simulink model "DFADAS2_SenFus_v1_201204RC_training_210115"  (R2018b)
settings: Solver=FixedStepDiscrete  StartTime=0.0  StopTime=inf  FixedStep=0.002  RelTol=1e-3  EnableMultiTasking=on
PreLoadFcn:
  | RTWConfigurationCB('preloadfcn', bdroot);
libraries: canmsglib x108, simulink x48, canfdmsglib x12
(part 27 of 28)

== system DFADAS2_SenFus_v1_201204RC_training_210115/Signal Input (Input)/Signal Input (10ms) (Input10)/VehInfo/Body Electric System State Receive and Processing (BESRx)/Steering Lamp CAN Frame PreProcess (StLampCANFrmPPrcs)/CAN Diagnosis (CANDia)/CheckSum Diagnosis (ChkSumDia)/Bit Check(BChk)/Bit Operating (BOp) ==
  note: CheckSum Error Flag Discription:
      | 1 : Fault
      | 0 : Normal
  note: Checksum Preprocess -- ChksumPre
  BOp_bByte0 : Inport
  BOp_bByte1 : Inport  Port=2
  BOp_bByte2 : Inport  Port=3
  BOp_bByte3 : Inport  Port=4
  BOp_bByte4 : Inport  Port=5
  BOp_bByte5 : Inport  Port=6
  BOp_bByte6 : Inport  Port=7
  BOp_bByte7 : Inport  Port=8
  Add : Sum  Inputs=+++++++
  Add1 : Sum  Inputs=+-
  Add2 : Sum  Inputs=+-
  ChksumPre1 : Subsystem
  ChksumPre2 : Subsystem
  ChksumPre3 : Subsystem
  ChksumPre4 : Subsystem
  ChksumPre5 : Subsystem
  ChksumPre6 : Subsystem
  ChksumPre7 : Subsystem
  Constant : Constant  Value=256  OutDataTypeStr=uint16  SampleTime=-1
  Constant1 : Constant  Value=255  OutDataTypeStr=uint8  SampleTime=-1
  Constant2 : Constant  OutDataTypeStr=uint8  SampleTime=-1
  Constant3 : Constant  Value=0  OutDataTypeStr=uint8  SampleTime=-1
  Data Type Conversion6 : DataTypeConversion  OutDataTypeStr=uint8
  Math Function : Math  Operator=mod  OutputSignalType=real  SaturateOnIntegerOverflow=on
  Switch : Switch  Criteria=u2 ~= 0
  BOp_efChkSumErrFlg : Outport
  wires:
  Switch/1 -> BOp_efChkSumErrFlg/1
  Constant3/1 -> Switch/3
  Constant2/1 -> Switch/1
  BOp_bByte7/1 -> ChksumPre7/1(In1)
  ChksumPre7/1(Out1) -> Add/7
  ChksumPre6/1(Out1) -> Add/6
  BOp_bByte6/1 -> ChksumPre6/2(In2)
  BOp_bByte5/1 -> ChksumPre6/1(In1)
  ChksumPre5/1(Out1) -> Add/5
  BOp_bByte4/1 -> ChksumPre5/2(In2)
  BOp_bByte3/1 -> ChksumPre5/1(In1)
  ChksumPre4/1(Out1) -> Add/4
  BOp_bByte2/1 -> ChksumPre4/1(In1), ChksumPre3/1(In1), ChksumPre2/1(In1)
  ChksumPre1/1(Out1) -> Add/1
  BOp_bByte1/1 -> ChksumPre1/1(In1)
  Constant1/1 -> Add1/1
  Math Function/1 -> Data Type Conversion6/1
  Constant/1 -> Math Function/2
  Add/1 -> Math Function/1
  Data Type Conversion6/1 -> Add1/2
  ChksumPre2/1(Out1) -> Add/2
  ChksumPre3/1(Out1) -> Add/3
  BOp_bByte0/1 -> Add2/1
  Add1/1 -> Add2/2
  Add2/1 -> Switch/2

== system DFADAS2_SenFus_v1_201204RC_training_210115/Signal Input (Input)/Signal Input (10ms) (Input10)/VehInfo/Function Keys State Receive and Processing (FKeyStRx)/Key Enable CAN Frame PreProcess (KeyEnaCANFrmPPrcs)/CAN Diagnosis (CANDia)/CheckSum Diagnosis (ChkSumDia)/Bit Check(BChk)/Bit Operating (BOp) ==
  note: Checksum Preprocess -- ChksumPre
  note: CheckSum Error Flag Discription:
      | 1 : Fault
      | 0 : Normal
  BOp_bByte0 : Inport
  BOp_bByte1 : Inport  Port=2
  BOp_bByte2 : Inport  Port=3
  BOp_bByte3 : Inport  Port=4
  BOp_bByte4 : Inport  Port=5
  BOp_bByte5 : Inport  Port=6
  BOp_bByte6 : Inport  Port=7
  BOp_bByte7 : Inport  Port=8
  Add : Sum  Inputs=+++++++
  Add1 : Sum  Inputs=+-
  Add2 : Sum  Inputs=+-
  ChksumPre1 : Subsystem
  ChksumPre2 : Subsystem
  ChksumPre3 : Subsystem
  ChksumPre4 : Subsystem
  ChksumPre5 : Subsystem
  ChksumPre6 : Subsystem
  ChksumPre7 : Subsystem
  Constant : Constant  Value=256  OutDataTypeStr=uint16  SampleTime=-1
  Constant1 : Constant  Value=255  OutDataTypeStr=uint8  SampleTime=-1
  Constant2 : Constant  OutDataTypeStr=uint8  SampleTime=-1
  Constant3 : Constant  Value=0  OutDataTypeStr=uint8  SampleTime=-1
  Data Type Conversion6 : DataTypeConversion  OutDataTypeStr=uint8
  Math Function : Math  Operator=mod  OutputSignalType=real  SaturateOnIntegerOverflow=on
  Switch : Switch  Criteria=u2 ~= 0
  BOp_efChkSumErrFlg : Outport
  wires:
  Add2/1 -> Switch/2
  Add1/1 -> Add2/2
  BOp_bByte0/1 -> Add2/1
  ChksumPre3/1(Out1) -> Add/3
  ChksumPre2/1(Out1) -> Add/2
  Data Type Conversion6/1 -> Add1/2
  Add/1 -> Math Function/1
  Constant/1 -> Math Function/2
  Math Function/1 -> Data Type Conversion6/1
  Constant1/1 -> Add1/1
  BOp_bByte1/1 -> ChksumPre1/1(In1)
  ChksumPre1/1(Out1) -> Add/1
  BOp_bByte2/1 -> ChksumPre2/1(In1), ChksumPre3/1(In1), ChksumPre4/1(In1)
  ChksumPre4/1(Out1) -> Add/4
  BOp_bByte3/1 -> ChksumPre5/1(In1)
  BOp_bByte4/1 -> ChksumPre5/2(In2)
  ChksumPre5/1(Out1) -> Add/5
  BOp_bByte5/1 -> ChksumPre6/1(In1)
  BOp_bByte6/1 -> ChksumPre6/2(In2)
  ChksumPre6/1(Out1) -> Add/6
  ChksumPre7/1(Out1) -> Add/7
  BOp_bByte7/1 -> ChksumPre7/1(In1)
  Constant2/1 -> Switch/1
  Constant3/1 -> Switch/3
  Switch/1 -> BOp_efChkSumErrFlg/1

== system DFADAS2_SenFus_v1_201204RC_training_210115/Signal Input (Input)/Signal Input (10ms) (Input10)/VehInfo/MP5 Signal Receive (MP5Rx)1/CAN Diagnosis (CANDia)/CheckSum Diagnosis (ChkSumDia)/Bit Check(BChk)/Bit Operating (BOp)/ChksumPre1 ==
  In1 : Inport
  Data Type Conversion7 : DataTypeConversion  OutDataTypeStr=uint16
  Out1 : Outport
  wires:
  Data Type Conversion7/1 -> Out1/1
  In1/1 -> Data Type Conversion7/1

== system DFADAS2_SenFus_v1_201204RC_training_210115/Signal Input (Input)/Signal Input (10ms) (Input10)/VehInfo/MP5 Signal Receive (MP5Rx)1/CAN Diagnosis (CANDia)/CheckSum Diagnosis (ChkSumDia)/Bit Check(BChk)/Bit Operating (BOp)/ChksumPre2 ==
  In1 : Inport
  Data Type Conversion7 : DataTypeConversion  OutDataTypeStr=uint16
  Extract Bits : simulink/Logic and Bit Operations/Extract Bits  bitsToExtract=Range of bits  numBits=8  bitIdxRange=6  outScalingMode=Treat bit field as an integer
      settings: SourceProductName=Simulink
  Out1 : Outport
  wires:
  Extract Bits/1 -> Data Type Conversion7/1
  In1/1 -> Extract Bits/1
  Data Type Conversion7/1 -> Out1/1

== system DFADAS2_SenFus_v1_201204RC_training_210115/Signal Input (Input)/Signal Input (10ms) (Input10)/VehInfo/MP5 Signal Receive (MP5Rx)1/CAN Diagnosis (CANDia)/CheckSum Diagnosis (ChkSumDia)/Bit Check(BChk)/Bit Operating (BOp)/ChksumPre3 ==
  In1 : Inport
  Data Type Conversion8 : DataTypeConversion  OutDataTypeStr=uint16
  Extract Bits1 : simulink/Logic and Bit Operations/Extract Bits  bitsToExtract=Range of bits  numBits=8  bitIdxRange=5  outScalingMode=Treat bit field as an integer
      settings: SourceProductName=Simulink
  Out1 : Outport
  wires:
  Extract Bits1/1 -> Data Type Conversion8/1
  In1/1 -> Extract Bits1/1
  Data Type Conversion8/1 -> Out1/1

== system DFADAS2_SenFus_v1_201204RC_training_210115/Signal Input (Input)/Signal Input (10ms) (Input10)/VehInfo/MP5 Signal Receive (MP5Rx)1/CAN Diagnosis (CANDia)/CheckSum Diagnosis (ChkSumDia)/Bit Check(BChk)/Bit Operating (BOp)/ChksumPre4 ==
  In1 : Inport
  Data Type Conversion8 : DataTypeConversion  OutDataTypeStr=uint16
  Extract Bits1 : simulink/Logic and Bit Operations/Extract Bits  bitsToExtract=Range of bits  numBits=8  bitIdxRange=4  outScalingMode=Treat bit field as an integer
      settings: SourceProductName=Simulink
  Out1 : Outport
  wires:
  Data Type Conversion8/1 -> Out1/1
  In1/1 -> Extract Bits1/1
  Extract Bits1/1 -> Data Type Conversion8/1

== system DFADAS2_SenFus_v1_201204RC_training_210115/Signal Input (Input)/Signal Input (10ms) (Input10)/VehInfo/MP5 Signal Receive (MP5Rx)1/CAN Diagnosis (CANDia)/CheckSum Diagnosis (ChkSumDia)/Bit Check(BChk)/Bit Operating (BOp)/ChksumPre5 ==
  In1 : Inport
  In2 : Inport  Port=2
  Add : Sum
  Data Type Conversion1 : DataTypeConversion  OutDataTypeStr=uint16
  Data Type Conversion4 : DataTypeConversion  OutDataTypeStr=uint16
  Shift Arithmetic2 : ArithShift  BitShiftNumber=-8
  Out1 : Outport
  wires:
  Data Type Conversion1/1 -> Add/2
  Data Type Conversion4/1 -> Shift Arithmetic2/1
  Add/1 -> Out1/1
  Shift Arithmetic2/1 -> Add/1
  In2/1 -> Data Type Conversion1/1
  In1/1 -> Data Type Conversion4/1

== system DFADAS2_SenFus_v1_201204RC_training_210115/Signal Input (Input)/Signal Input (10ms) (Input10)/VehInfo/MP5 Signal Receive (MP5Rx)1/CAN Diagnosis (CANDia)/CheckSum Diagnosis (ChkSumDia)/Bit Check(BChk)/Bit Operating (BOp)/ChksumPre6 ==
  In1 : Inport
  In2 : Inport  Port=2
  Add : Sum
  Data Type Conversion1 : DataTypeConversion  OutDataTypeStr=uint16
  Data Type Conversion4 : DataTypeConversion  OutDataTypeStr=uint16
  Shift Arithmetic2 : ArithShift  BitShiftNumber=-8
  Out1 : Outport
  wires:
  In1/1 -> Data Type Conversion4/1
  In2/1 -> Data Type Conversion1/1
  Shift Arithmetic2/1 -> Add/1
  Add/1 -> Out1/1
  Data Type Conversion4/1 -> Shift Arithmetic2/1
  Data Type Conversion1/1 -> Add/2

== system DFADAS2_SenFus_v1_201204RC_training_210115/Signal Input (Input)/Signal Input (10ms) (Input10)/VehInfo/MP5 Signal Receive (MP5Rx)1/CAN Diagnosis (CANDia)/CheckSum Diagnosis (ChkSumDia)/Bit Check(BChk)/Bit Operating (BOp)/ChksumPre7 ==
  In1 : Inport
  Data Type Conversion8 : DataTypeConversion  OutDataTypeStr=uint16
  Extract Bits1 : simulink/Logic and Bit Operations/Extract Bits  bitsToExtract=Range of bits  numBits=8  bitIdxRange=7  outScalingMode=Treat bit field as an integer
      settings: SourceProductName=Simulink
  Out1 : Outport
  wires:
  Extract Bits1/1 -> Data Type Conversion8/1
  In1/1 -> Extract Bits1/1
  Data Type Conversion8/1 -> Out1/1

== system DFADAS2_SenFus_v1_201204RC_training_210115/Signal Input (Input)/Signal Input (10ms) (Input10)/VehInfo/Vehicle Movement Signal Receive and Processing (VehMovRx)/VehSpd CAN Frame PreProcess (VehSpdCANFrmPPrcs)/CAN Diagnosis (CANDia)/CheckSum Diagnosis (ChkSumDia)/Bit Check(BChk)/Bit Operating (BOp) ==
  note: Checksum Preprocess -- ChksumPre
  note: CheckSum Error Flag Discription:
      | 1 : Fault
      | 0 : Normal
  BOp_bByte0 : Inport
  BOp_bByte1 : Inport  Port=2
  BOp_bByte2 : Inport  Port=3
  BOp_bByte3 : Inport  Port=4
  BOp_bByte4 : Inport  Port=5
  BOp_bByte5 : Inport  Port=6
  BOp_bByte6 : Inport  Port=7
  BOp_bByte7 : Inport  Port=8
  Add : Sum  Inputs=+++++++
  Add1 : Sum  Inputs=+-
  Add2 : Sum  Inputs=+-
  ChksumPre1 : Subsystem
  ChksumPre2 : Subsystem
  ChksumPre3 : Subsystem
  ChksumPre4 : Subsystem
  ChksumPre5 : Subsystem
  ChksumPre6 : Subsystem
  ChksumPre7 : Subsystem
  Constant : Constant  Value=256  OutDataTypeStr=uint16  SampleTime=-1
  Constant1 : Constant  Value=255  OutDataTypeStr=uint8  SampleTime=-1
  Constant2 : Constant  OutDataTypeStr=uint8  SampleTime=-1
  Constant3 : Constant  Value=0  OutDataTypeStr=uint8  SampleTime=-1
  Data Type Conversion6 : DataTypeConversion  OutDataTypeStr=uint8
  Math Function : Math  Operator=mod  OutputSignalType=real  SaturateOnIntegerOverflow=on
  Switch : Switch  Criteria=u2 ~= 0
  BOp_efChkSumErrFlg : Outport
  wires:
  Add2/1 -> Switch/2
  Add1/1 -> Add2/2
  BOp_bByte0/1 -> Add2/1
  ChksumPre3/1(Out1) -> Add/3
  ChksumPre2/1(Out1) -> Add/2
  Data Type Conversion6/1 -> Add1/2
  Add/1 -> Math Function/1
  Constant/1 -> Math Function/2
  Math Function/1 -> Data Type Conversion6/1
  Constant1/1 -> Add1/1
  BOp_bByte1/1 -> ChksumPre1/1(In1)
  ChksumPre1/1(Out1) -> Add/1
  BOp_bByte2/1 -> ChksumPre2/1(In1), ChksumPre3/1(In1), ChksumPre4/1(In1)
  ChksumPre4/1(Out1) -> Add/4
  BOp_bByte3/1 -> ChksumPre5/1(In1)
  BOp_bByte4/1 -> ChksumPre5/2(In2)
  ChksumPre5/1(Out1) -> Add/5
  BOp_bByte5/1 -> ChksumPre6/1(In1)
  BOp_bByte6/1 -> ChksumPre6/2(In2)
  ChksumPre6/1(Out1) -> Add/6
  ChksumPre7/1(Out1) -> Add/7
  BOp_bByte7/1 -> ChksumPre7/1(In1)
  Constant2/1 -> Switch/1
  Constant3/1 -> Switch/3
  Switch/1 -> BOp_efChkSumErrFlg/1

== system DFADAS2_SenFus_v1_201204RC_training_210115/Signal Input (Input)/Signal Input (10ms) (Input10)/VehInfo/Vehicle Movement Signal Receive and Processing (VehMovRx)/Yaw State CAN Frame PreProcess (YawCANFrmPPrcs)/CAN Diagnosis (CANDia)/CheckSum Diagnosis (ChkSumDia)/Bit Check(BChk)/Bit Operating (BOp) ==
  note: Checksum Preprocess -- ChksumPre
  note: CheckSum Error Flag Discription:
      | 1 : Fault
      | 0 : Normal
  BOp_bByte0 : Inport
  BOp_bByte1 : Inport  Port=2
  BOp_bByte2 : Inport  Port=3
  BOp_bByte3 : Inport  Port=4
  BOp_bByte4 : Inport  Port=5
  BOp_bByte5 : Inport  Port=6
  BOp_bByte6 : Inport  Port=7
  BOp_bByte7 : Inport  Port=8
  Add : Sum  Inputs=+++++++
  Add1 : Sum  Inputs=+-
  Add2 : Sum  Inputs=+-
  ChksumPre1 : Subsystem
  ChksumPre2 : Subsystem
  ChksumPre3 : Subsystem
  ChksumPre4 : Subsystem
  ChksumPre5 : Subsystem
  ChksumPre6 : Subsystem
  ChksumPre7 : Subsystem
  Constant : Constant  Value=256  OutDataTypeStr=uint16  SampleTime=-1
  Constant1 : Constant  Value=255  OutDataTypeStr=uint8  SampleTime=-1
  Constant2 : Constant  OutDataTypeStr=uint8  SampleTime=-1
  Constant3 : Constant  Value=0  OutDataTypeStr=uint8  SampleTime=-1
  Data Type Conversion6 : DataTypeConversion  OutDataTypeStr=uint8
  Math Function : Math  Operator=mod  OutputSignalType=real  SaturateOnIntegerOverflow=on
  Switch : Switch  Criteria=u2 ~= 0
  BOp_efChkSumErrFlg : Outport
  wires:
  Add2/1 -> Switch/2
  Add1/1 -> Add2/2
  BOp_bByte0/1 -> Add2/1
  ChksumPre3/1(Out1) -> Add/3
  ChksumPre2/1(Out1) -> Add/2
  Data Type Conversion6/1 -> Add1/2
  Add/1 -> Math Function/1
  Constant/1 -> Math Function/2
  Math Function/1 -> Data Type Conversion6/1
  Constant1/1 -> Add1/1
  BOp_bByte1/1 -> ChksumPre1/1(In1)
  ChksumPre1/1(Out1) -> Add/1
  BOp_bByte2/1 -> ChksumPre2/1(In1), ChksumPre3/1(In1), ChksumPre4/1(In1)
  ChksumPre4/1(Out1) -> Add/4
  BOp_bByte3/1 -> ChksumPre5/1(In1)
  BOp_bByte4/1 -> ChksumPre5/2(In2)
  ChksumPre5/1(Out1) -> Add/5
  BOp_bByte5/1 -> ChksumPre6/1(In1)
  BOp_bByte6/1 -> ChksumPre6/2(In2)
  ChksumPre6/1(Out1) -> Add/6
  ChksumPre7/1(Out1) -> Add/7
  BOp_bByte7/1 -> ChksumPre7/1(In1)
  Constant2/1 -> Switch/1
  Constant3/1 -> Switch/3
  Switch/1 -> BOp_efChkSumErrFlg/1

== system DFADAS2_SenFus_v1_201204RC_training_210115/Signal Input (Input)/Signal Input (50ms) (Input50)/Cmr/CmrInfo/L0 Information (L0Info) /CAN Diagnosis (CANDia)1/CheckSum Diagnosis (ChkSumDia)/Bit Check(BChk)/Bit Operating (BOp) ==
  note: Checksum Preprocess -- ChksumPre
  note: CheckSum Error Flag Discription:
      | 1 : Fault
      | 0 : Normal
  Chksum in Frame : Inport
  BOp_bByte1 : Inport  Port=2
  BOp_bByte2 : Inport  Port=3
  BOp_bByte3 : Inport  Port=4
  BOp_bByte4 : Inport  Port=5
  BOp_bByte5 : Inport  Port=6
  BOp_bByte6 : Inport  Port=7
  BOp_bByte7 : Inport  Port=8
  Add : Sum  Inputs=+++++++
  Add1 : Sum  Inputs=+-
  Add2 : Sum  Inputs=+-
  ChksumPre1 : Subsystem
  ChksumPre2 : Subsystem
  ChksumPre3 : Subsystem
  ChksumPre4 : Subsystem
  ChksumPre5 : Subsystem
  ChksumPre6 : Subsystem
  ChksumPre7 : Subsystem
  Constant : Constant  Value=256  OutDataTypeStr=uint16  SampleTime=-1
  Constant1 : Constant  Value=255  OutDataTypeStr=uint8  SampleTime=-1
  Constant2 : Constant  OutDataTypeStr=uint8  SampleTime=-1
  Constant3 : Constant  Value=0  OutDataTypeStr=uint8  SampleTime=-1
  Data Type Conversion6 : DataTypeConversion  OutDataTypeStr=uint8
  Math Function : Math  Operator=mod  OutputSignalType=real  SaturateOnIntegerOverflow=on
  Switch : Switch  Criteria=u2 ~= 0
  BOp_efChkSumErrFlg : Outport
  wires:
  Add2/1 -> Switch/2
  Add1/1 -> Add2/2
  Chksum in Frame/1 -> Add2/1
  ChksumPre3/1(Out1) -> Add/3
  ChksumPre2/1(Out1) -> Add/2
  Data Type Conversion6/1 -> Add1/2
  Add/1 -> Math Function/1
  Constant/1 -> Math Function/2
  Math Function/1 -> Data Type Conversion6/1
  Constant1/1 -> Add1/1
  BOp_bByte1/1 -> ChksumPre1/1(In1)
  ChksumPre1/1(Out1) -> Add/1
  BOp_bByte2/1 -> ChksumPre2/1(In1), ChksumPre3/1(In1), ChksumPre4/1(In1)
  ChksumPre4/1(Out1) -> Add/4
  BOp_bByte3/1 -> ChksumPre5/1(In1)
  BOp_bByte4/1 -> ChksumPre5/2(In2)
  ChksumPre5/1(Out1) -> Add/5
  BOp_bByte5/1 -> ChksumPre6/1(In1)
  BOp_bByte6/1 -> ChksumPre6/2(In2)
  ChksumPre6/1(Out1) -> Add/6
  ChksumPre7/1(Out1) -> Add/7
  BOp_bByte7/1 -> ChksumPre7/1(In1)
  Constant2/1 -> Switch/1
  Constant3/1 -> Switch/3
  Switch/1 -> BOp_efChkSumErrFlg/1

== system DFADAS2_SenFus_v1_201204RC_training_210115/Signal Input (Input)/Signal Input (50ms) (Input50)/Cmr/CmrInfo/L1 Information (L1Info)/CAN Diagnosis (CANDia)/CheckSum Diagnosis (ChkSumDia)/Bit Check(BChk)/Bit Operating (BOp) ==
  note: Checksum Preprocess -- ChksumPre
  note: CheckSum Error Flag Discription:
      | 1 : Fault
      | 0 : Normal
  Chksum in Frame : Inport
  BOp_bByte1 : Inport  Port=2
  BOp_bByte2 : Inport  Port=3
  BOp_bByte3 : Inport  Port=4
  BOp_bByte4 : Inport  Port=5
  BOp_bByte5 : Inport  Port=6
  BOp_bByte6 : Inport  Port=7
  BOp_bByte7 : Inport  Port=8
  Add : Sum  Inputs=+++++++
  Add1 : Sum  Inputs=+-
  Add2 : Sum  Inputs=+-
  ChksumPre1 : Subsystem
  ChksumPre2 : Subsystem
  ChksumPre3 : Subsystem
  ChksumPre4 : Subsystem
  ChksumPre5 : Subsystem
  ChksumPre6 : Subsystem
  ChksumPre7 : Subsystem
  Constant : Constant  Value=256  OutDataTypeStr=uint16  SampleTime=-1
  Constant1 : Constant  Value=255  OutDataTypeStr=uint8  SampleTime=-1
  Constant2 : Constant  OutDataTypeStr=uint8  SampleTime=-1
  Constant3 : Constant  Value=0  OutDataTypeStr=uint8  SampleTime=-1
  Data Type Conversion6 : DataTypeConversion  OutDataTypeStr=uint8
  Math Function : Math  Operator=mod  OutputSignalType=real  SaturateOnIntegerOverflow=on
  Switch : Switch  Criteria=u2 ~= 0
  BOp_efChkSumErrFlg : Outport
  wires:
  Add2/1 -> Switch/2
  Add1/1 -> Add2/2
  Chksum in Frame/1 -> Add2/1
  ChksumPre3/1(Out1) -> Add/3
  ChksumPre2/1(Out1) -> Add/2
  Data Type Conversion6/1 -> Add1/2
  Add/1 -> Math Function/1
  Constant/1 -> Math Function/2
  Math Function/1 -> Data Type Conversion6/1
  Constant1/1 -> Add1/1
  BOp_bByte1/1 -> ChksumPre1/1(In1)
  ChksumPre1/1(Out1) -> Add/1
  BOp_bByte2/1 -> ChksumPre2/1(In1), ChksumPre3/1(In1), ChksumPre4/1(In1)
  ChksumPre4/1(Out1) -> Add/4
  BOp_bByte3/1 -> ChksumPre5/1(In1)
  BOp_bByte4/1 -> ChksumPre5/2(In2)
  ChksumPre5/1(Out1) -> Add/5
  BOp_bByte5/1 -> ChksumPre6/1(In1)
  BOp_bByte6/1 -> ChksumPre6/2(In2)
  ChksumPre6/1(Out1) -> Add/6
  ChksumPre7/1(Out1) -> Add/7
  BOp_bByte7/1 -> ChksumPre7/1(In1)
  Constant2/1 -> Switch/1
  Constant3/1 -> Switch/3
  Switch/1 -> BOp_efChkSumErrFlg/1

== system DFADAS2_SenFus_v1_201204RC_training_210115/Signal Input (Input)/Signal Input (50ms) (Input50)/Cmr/CmrInfo/R0 Information (R0Info)/CAN Diagnosis (CANDia)/CheckSum Diagnosis (ChkSumDia)/Bit Check(BChk)/Bit Operating (BOp) ==
  note: Checksum Preprocess -- ChksumPre
  note: CheckSum Error Flag Discription:
      | 1 : Fault
      | 0 : Normal
  Chksum in Frame : Inport
  BOp_bByte1 : Inport  Port=2
  BOp_bByte2 : Inport  Port=3
  BOp_bByte3 : Inport  Port=4
  BOp_bByte4 : Inport  Port=5
  BOp_bByte5 : Inport  Port=6
  BOp_bByte6 : Inport  Port=7
  BOp_bByte7 : Inport  Port=8
  Add : Sum  Inputs=+++++++
  Add1 : Sum  Inputs=+-
  Add2 : Sum  Inputs=+-
  ChksumPre1 : Subsystem
  ChksumPre2 : Subsystem
  ChksumPre3 : Subsystem
  ChksumPre4 : Subsystem
  ChksumPre5 : Subsystem
  ChksumPre6 : Subsystem
  ChksumPre7 : Subsystem
  Constant : Constant  Value=256  OutDataTypeStr=uint16  SampleTime=-1
  Constant1 : Constant  Value=255  OutDataTypeStr=uint8  SampleTime=-1
  Constant2 : Constant  OutDataTypeStr=uint8  SampleTime=-1
  Constant3 : Constant  Value=0  OutDataTypeStr=uint8  SampleTime=-1
  Data Type Conversion6 : DataTypeConversion  OutDataTypeStr=uint8
  Math Function : Math  Operator=mod  OutputSignalType=real  SaturateOnIntegerOverflow=on
  Switch : Switch  Criteria=u2 ~= 0
  BOp_efChkSumErrFlg : Outport
  wires:
  Add2/1 -> Switch/2
  Add1/1 -> Add2/2
  Chksum in Frame/1 -> Add2/1
  ChksumPre3/1(Out1) -> Add/3
  ChksumPre2/1(Out1) -> Add/2
  Data Type Conversion6/1 -> Add1/2
  Add/1 -> Math Function/1
  Constant/1 -> Math Function/2
  Math Function/1 -> Data Type Conversion6/1
  Constant1/1 -> Add1/1
  BOp_bByte1/1 -> ChksumPre1/1(In1)
  ChksumPre1/1(Out1) -> Add/1
  BOp_bByte2/1 -> ChksumPre2/1(In1), ChksumPre3/1(In1), ChksumPre4/1(In1)
  ChksumPre4/1(Out1) -> Add/4
  BOp_bByte3/1 -> ChksumPre5/1(In1)
  BOp_bByte4/1 -> ChksumPre5/2(In2)
  ChksumPre5/1(Out1) -> Add/5
  BOp_bByte5/1 -> ChksumPre6/1(In1)
  BOp_bByte6/1 -> ChksumPre6/2(In2)
  ChksumPre6/1(Out1) -> Add/6
  ChksumPre7/1(Out1) -> Add/7
  BOp_bByte7/1 -> ChksumPre7/1(In1)
  Constant2/1 -> Switch/1
  Constant3/1 -> Switch/3
  Switch/1 -> BOp_efChkSumErrFlg/1

== system DFADAS2_SenFus_v1_201204RC_training_210115/Signal Input (Input)/Signal Input (50ms) (Input50)/Cmr/CmrInfo/R1 Information (R1Info)/CAN Diagnosis (CANDia)/CheckSum Diagnosis (ChkSumDia)/Bit Check(BChk)/Bit Operating (BOp) ==
  note: CheckSum Error Flag Discription:
      | 1 : Fault
      | 0 : Normal
  note: Checksum Preprocess -- ChksumPre
  Chksum in Frame : Inport
  BOp_bByte1 : Inport  Port=2
  BOp_bByte2 : Inport  Port=3
  BOp_bByte3 : Inport  Port=4
  BOp_bByte4 : Inport  Port=5
  BOp_bByte5 : Inport  Port=6
  BOp_bByte6 : Inport  Port=7
  BOp_bByte7 : Inport  Port=8
  Add : Sum  Inputs=+++++++
  Add1 : Sum  Inputs=+-
  Add2 : Sum  Inputs=+-
  ChksumPre1 : Subsystem
  ChksumPre2 : Subsystem
  ChksumPre3 : Subsystem
  ChksumPre4 : Subsystem
  ChksumPre5 : Subsystem
  ChksumPre6 : Subsystem
  ChksumPre7 : Subsystem
  Constant : Constant  Value=256  OutDataTypeStr=uint16  SampleTime=-1
  Constant1 : Constant  Value=255  OutDataTypeStr=uint8  SampleTime=-1
  Constant2 : Constant  OutDataTypeStr=uint8  SampleTime=-1
  Constant3 : Constant  Value=0  OutDataTypeStr=uint8  SampleTime=-1
  Data Type Conversion6 : DataTypeConversion  OutDataTypeStr=uint8
  Math Function : Math  Operator=mod  OutputSignalType=real  SaturateOnIntegerOverflow=on
  Switch : Switch  Criteria=u2 ~= 0
  BOp_efChkSumErrFlg : Outport
  wires:
  Switch/1 -> BOp_efChkSumErrFlg/1
  Constant3/1 -> Switch/3
  Constant2/1 -> Switch/1
  BOp_bByte7/1 -> ChksumPre7/1(In1)
  ChksumPre7/1(Out1) -> Add/7
  ChksumPre6/1(Out1) -> Add/6
  BOp_bByte6/1 -> ChksumPre6/2(In2)
  BOp_bByte5/1 -> ChksumPre6/1(In1)
  ChksumPre5/1(Out1) -> Add/5
  BOp_bByte4/1 -> ChksumPre5/2(In2)
  BOp_bByte3/1 -> ChksumPre5/1(In1)
  ChksumPre4/1(Out1) -> Add/4
  BOp_bByte2/1 -> ChksumPre4/1(In1), ChksumPre3/1(In1), ChksumPre2/1(In1)
  ChksumPre1/1(Out1) -> Add/1
  BOp_bByte1/1 -> ChksumPre1/1(In1)
  Constant1/1 -> Add1/1
  Math Function/1 -> Data Type Conversion6/1
  Constant/1 -> Math Function/2
  Add/1 -> Math Function/1
  Data Type Conversion6/1 -> Add1/2
  ChksumPre2/1(Out1) -> Add/2
  ChksumPre3/1(Out1) -> Add/3
  Chksum in Frame/1 -> Add2/1
  Add1/1 -> Add2/2
  Add2/1 -> Switch/2

== system DFADAS2_SenFus_v1_201204RC_training_210115/Signal Input (Input)/Signal Input (10ms) (Input10)/VehInfo/Body Electric System State Receive and Processing (BESRx)/Steering Lamp CAN Frame PreProcess (StLampCANFrmPPrcs)/CAN Diagnosis (CANDia)/CheckSum Diagnosis (ChkSumDia)/Bit Check(BChk)/Bit Operating (BOp)/ChksumPre1 ==
  In1 : Inport
  Data Type Conversion7 : DataTypeConversion  OutDataTypeStr=uint16
  Out1 : Outport
  wires:
  Data Type Conversion7/1 -> Out1/1
  In1/1 -> Data Type Conversion7/1

== system DFADAS2_SenFus_v1_201204RC_training_210115/Signal Input (Input)/Signal Input (10ms) (Input10)/VehInfo/Body Electric System State Receive and Processing (BESRx)/Steering Lamp CAN Frame PreProcess (StLampCANFrmPPrcs)/CAN Diagnosis (CANDia)/CheckSum Diagnosis (ChkSumDia)/Bit Check(BChk)/Bit Operating (BOp)/ChksumPre2 ==
  In1 : Inport
  Data Type Conversion7 : DataTypeConversion  OutDataTypeStr=uint16
  Extract Bits : simulink/Logic and Bit Operations/Extract Bits  bitsToExtract=Range of bits  numBits=8  bitIdxRange=6  outScalingMode=Treat bit field as an integer
      settings: SourceProductName=Simulink
  Out1 : Outport
  wires:
  Extract Bits/1 -> Data Type Conversion7/1
  In1/1 -> Extract Bits/1
  Data Type Conversion7/1 -> Out1/1

== system DFADAS2_SenFus_v1_201204RC_training_210115/Signal Input (Input)/Signal Input (10ms) (Input10)/VehInfo/Body Electric System State Receive and Processing (BESRx)/Steering Lamp CAN Frame PreProcess (StLampCANFrmPPrcs)/CAN Diagnosis (CANDia)/CheckSum Diagnosis (ChkSumDia)/Bit Check(BChk)/Bit Operating (BOp)/ChksumPre3 ==
  In1 : Inport
  Data Type Conversion8 : DataTypeConversion  OutDataTypeStr=uint16
  Extract Bits1 : simulink/Logic and Bit Operations/Extract Bits  bitsToExtract=Range of bits  numBits=8  bitIdxRange=5  outScalingMode=Treat bit field as an integer
      settings: SourceProductName=Simulink
  Out1 : Outport
  wires:
  Extract Bits1/1 -> Data Type Conversion8/1
  In1/1 -> Extract Bits1/1
  Data Type Conversion8/1 -> Out1/1

== system DFADAS2_SenFus_v1_201204RC_training_210115/Signal Input (Input)/Signal Input (10ms) (Input10)/VehInfo/Body Electric System State Receive and Processing (BESRx)/Steering Lamp CAN Frame PreProcess (StLampCANFrmPPrcs)/CAN Diagnosis (CANDia)/CheckSum Diagnosis (ChkSumDia)/Bit Check(BChk)/Bit Operating (BOp)/ChksumPre4 ==
  In1 : Inport
  Data Type Conversion8 : DataTypeConversion  OutDataTypeStr=uint16
  Extract Bits1 : simulink/Logic and Bit Operations/Extract Bits  bitsToExtract=Range of bits  numBits=8  bitIdxRange=4  outScalingMode=Treat bit field as an integer
      settings: SourceProductName=Simulink
  Out1 : Outport
  wires:
  Data Type Conversion8/1 -> Out1/1
  In1/1 -> Extract Bits1/1
  Extract Bits1/1 -> Data Type Conversion8/1

== system DFADAS2_SenFus_v1_201204RC_training_210115/Signal Input (Input)/Signal Input (10ms) (Input10)/VehInfo/Body Electric System State Receive and Processing (BESRx)/Steering Lamp CAN Frame PreProcess (StLampCANFrmPPrcs)/CAN Diagnosis (CANDia)/CheckSum Diagnosis (ChkSumDia)/Bit Check(BChk)/Bit Operating (BOp)/ChksumPre5 ==
  In1 : Inport
  In2 : Inport  Port=2
  Add : Sum
  Data Type Conversion1 : DataTypeConversion  OutDataTypeStr=uint16
  Data Type Conversion4 : DataTypeConversion  OutDataTypeStr=uint16
  Shift Arithmetic2 : ArithShift  BitShiftNumber=-8
  Out1 : Outport
  wires:
  Data Type Conversion1/1 -> Add/2
  Data Type Conversion4/1 -> Shift Arithmetic2/1
  Add/1 -> Out1/1
  Shift Arithmetic2/1 -> Add/1
  In2/1 -> Data Type Conversion1/1
  In1/1 -> Data Type Conversion4/1

== system DFADAS2_SenFus_v1_201204RC_training_210115/Signal Input (Input)/Signal Input (10ms) (Input10)/VehInfo/Body Electric System State Receive and Processing (BESRx)/Steering Lamp CAN Frame PreProcess (StLampCANFrmPPrcs)/CAN Diagnosis (CANDia)/CheckSum Diagnosis (ChkSumDia)/Bit Check(BChk)/Bit Operating (BOp)/ChksumPre6 ==
  In1 : Inport
  In2 : Inport  Port=2
  Add : Sum
  Data Type Conversion1 : DataTypeConversion  OutDataTypeStr=uint16
  Data Type Conversion4 : DataTypeConversion  OutDataTypeStr=uint16
  Shift Arithmetic2 : ArithShift  BitShiftNumber=-8
  Out1 : Outport
  wires:
  In1/1 -> Data Type Conversion4/1
  In2/1 -> Data Type Conversion1/1
  Shift Arithmetic2/1 -> Add/1
  Add/1 -> Out1/1
  Data Type Conversion4/1 -> Shift Arithmetic2/1
  Data Type Conversion1/1 -> Add/2

== system DFADAS2_SenFus_v1_201204RC_training_210115/Signal Input (Input)/Signal Input (10ms) (Input10)/VehInfo/Body Electric System State Receive and Processing (BESRx)/Steering Lamp CAN Frame PreProcess (StLampCANFrmPPrcs)/CAN Diagnosis (CANDia)/CheckSum Diagnosis (ChkSumDia)/Bit Check(BChk)/Bit Operating (BOp)/ChksumPre7 ==
  In1 : Inport
  Data Type Conversion8 : DataTypeConversion  OutDataTypeStr=uint16
  Extract Bits1 : simulink/Logic and Bit Operations/Extract Bits  bitsToExtract=Range of bits  numBits=8  bitIdxRange=7  outScalingMode=Treat bit field as an integer
      settings: SourceProductName=Simulink
  Out1 : Outport
  wires:
  Extract Bits1/1 -> Data Type Conversion8/1
  In1/1 -> Extract Bits1/1
  Data Type Conversion8/1 -> Out1/1

== system DFADAS2_SenFus_v1_201204RC_training_210115/Signal Input (Input)/Signal Input (10ms) (Input10)/VehInfo/Function Keys State Receive and Processing (FKeyStRx)/Key Enable CAN Frame PreProcess (KeyEnaCANFrmPPrcs)/CAN Diagnosis (CANDia)/CheckSum Diagnosis (ChkSumDia)/Bit Check(BChk)/Bit Operating (BOp)/ChksumPre1 ==
  In1 : Inport
  Data Type Conversion7 : DataTypeConversion  OutDataTypeStr=uint16
  Out1 : Outport
  wires:
  In1/1 -> Data Type Conversion7/1
  Data Type Conversion7/1 -> Out1/1

== system DFADAS2_SenFus_v1_201204RC_training_210115/Signal Input (Input)/Signal Input (10ms) (Input10)/VehInfo/Function Keys State Receive and Processing (FKeyStRx)/Key Enable CAN Frame PreProcess (KeyEnaCANFrmPPrcs)/CAN Diagnosis (CANDia)/CheckSum Diagnosis (ChkSumDia)/Bit Check(BChk)/Bit Operating (BOp)/ChksumPre2 ==
  In1 : Inport
  Data Type Conversion7 : DataTypeConversion  OutDataTypeStr=uint16
  Extract Bits : simulink/Logic and Bit Operations/Extract Bits  bitsToExtract=Range of bits  numBits=8  bitIdxRange=6  outScalingMode=Treat bit field as an integer
      settings: SourceProductName=Simulink
  Out1 : Outport
  wires:
  Data Type Conversion7/1 -> Out1/1
  In1/1 -> Extract Bits/1
  Extract Bits/1 -> Data Type Conversion7/1

== system DFADAS2_SenFus_v1_201204RC_training_210115/Signal Input (Input)/Signal Input (10ms) (Input10)/VehInfo/Function Keys State Receive and Processing (FKeyStRx)/Key Enable CAN Frame PreProcess (KeyEnaCANFrmPPrcs)/CAN Diagnosis (CANDia)/CheckSum Diagnosis (ChkSumDia)/Bit Check(BChk)/Bit Operating (BOp)/ChksumPre3 ==
  In1 : Inport
  Data Type Conversion8 : DataTypeConversion  OutDataTypeStr=uint16
  Extract Bits1 : simulink/Logic and Bit Operations/Extract Bits  bitsToExtract=Range of bits  numBits=8  bitIdxRange=5  outScalingMode=Treat bit field as an integer
      settings: SourceProductName=Simulink
  Out1 : Outport
  wires:
  Data Type Conversion8/1 -> Out1/1
  In1/1 -> Extract Bits1/1
  Extract Bits1/1 -> Data Type Conversion8/1

== system DFADAS2_SenFus_v1_201204RC_training_210115/Signal Input (Input)/Signal Input (10ms) (Input10)/VehInfo/Function Keys State Receive and Processing (FKeyStRx)/Key Enable CAN Frame PreProcess (KeyEnaCANFrmPPrcs)/CAN Diagnosis (CANDia)/CheckSum Diagnosis (ChkSumDia)/Bit Check(BChk)/Bit Operating (BOp)/ChksumPre4 ==
  In1 : Inport
  Data Type Conversion8 : DataTypeConversion  OutDataTypeStr=uint16
  Extract Bits1 : simulink/Logic and Bit Operations/Extract Bits  bitsToExtract=Range of bits  numBits=8  bitIdxRange=4  outScalingMode=Treat bit field as an integer
      settings: SourceProductName=Simulink
  Out1 : Outport
  wires:
  Extract Bits1/1 -> Data Type Conversion8/1
  In1/1 -> Extract Bits1/1
  Data Type Conversion8/1 -> Out1/1

== system DFADAS2_SenFus_v1_201204RC_training_210115/Signal Input (Input)/Signal Input (10ms) (Input10)/VehInfo/Function Keys State Receive and Processing (FKeyStRx)/Key Enable CAN Frame PreProcess (KeyEnaCANFrmPPrcs)/CAN Diagnosis (CANDia)/CheckSum Diagnosis (ChkSumDia)/Bit Check(BChk)/Bit Operating (BOp)/ChksumPre5 ==
  In1 : Inport
  In2 : Inport  Port=2
  Add : Sum
  Data Type Conversion1 : DataTypeConversion  OutDataTypeStr=uint16
  Data Type Conversion4 : DataTypeConversion  OutDataTypeStr=uint16
  Shift Arithmetic2 : ArithShift  BitShiftNumber=-8
  Out1 : Outport
  wires:
  In1/1 -> Data Type Conversion4/1
  In2/1 -> Data Type Conversion1/1
  Shift Arithmetic2/1 -> Add/1
  Add/1 -> Out1/1
  Data Type Conversion4/1 -> Shift Arithmetic2/1
  Data Type Conversion1/1 -> Add/2

== system DFADAS2_SenFus_v1_201204RC_training_210115/Signal Input (Input)/Signal Input (10ms) (Input10)/VehInfo/Function Keys State Receive and Processing (FKeyStRx)/Key Enable CAN Frame PreProcess (KeyEnaCANFrmPPrcs)/CAN Diagnosis (CANDia)/CheckSum Diagnosis (ChkSumDia)/Bit Check(BChk)/Bit Operating (BOp)/ChksumPre6 ==
  In1 : Inport
  In2 : Inport  Port=2
  Add : Sum
  Data Type Conversion1 : DataTypeConversion  OutDataTypeStr=uint16
  Data Type Conversion4 : DataTypeConversion  OutDataTypeStr=uint16
  Shift Arithmetic2 : ArithShift  BitShiftNumber=-8
  Out1 : Outport
  wires:
  Data Type Conversion1/1 -> Add/2
  Data Type Conversion4/1 -> Shift Arithmetic2/1
  Add/1 -> Out1/1
  Shift Arithmetic2/1 -> Add/1
  In2/1 -> Data Type Conversion1/1
  In1/1 -> Data Type Conversion4/1

== system DFADAS2_SenFus_v1_201204RC_training_210115/Signal Input (Input)/Signal Input (10ms) (Input10)/VehInfo/Function Keys State Receive and Processing (FKeyStRx)/Key Enable CAN Frame PreProcess (KeyEnaCANFrmPPrcs)/CAN Diagnosis (CANDia)/CheckSum Diagnosis (ChkSumDia)/Bit Check(BChk)/Bit Operating (BOp)/ChksumPre7 ==
  In1 : Inport
  Data Type Conversion8 : DataTypeConversion  OutDataTypeStr=uint16
  Extract Bits1 : simulink/Logic and Bit Operations/Extract Bits  bitsToExtract=Range of bits  numBits=8  bitIdxRange=7  outScalingMode=Treat bit field as an integer
      settings: SourceProductName=Simulink
  Out1 : Outport
  wires:
  Data Type Conversion8/1 -> Out1/1
  In1/1 -> Extract Bits1/1
  Extract Bits1/1 -> Data Type Conversion8/1

== system DFADAS2_SenFus_v1_201204RC_training_210115/Signal Input (Input)/Signal Input (10ms) (Input10)/VehInfo/Vehicle Movement Signal Receive and Processing (VehMovRx)/VehSpd CAN Frame PreProcess (VehSpdCANFrmPPrcs)/CAN Diagnosis (CANDia)/CheckSum Diagnosis (ChkSumDia)/Bit Check(BChk)/Bit Operating (BOp)/ChksumPre1 ==
  In1 : Inport
  Data Type Conversion7 : DataTypeConversion  OutDataTypeStr=uint16
  Out1 : Outport
  wires:
  In1/1 -> Data Type Conversion7/1
  Data Type Conversion7/1 -> Out1/1

== system DFADAS2_SenFus_v1_201204RC_training_210115/Signal Input (Input)/Signal Input (10ms) (Input10)/VehInfo/Vehicle Movement Signal Receive and Processing (VehMovRx)/VehSpd CAN Frame PreProcess (VehSpdCANFrmPPrcs)/CAN Diagnosis (CANDia)/CheckSum Diagnosis (ChkSumDia)/Bit Check(BChk)/Bit Operating (BOp)/ChksumPre2 ==
  In1 : Inport
  Data Type Conversion7 : DataTypeConversion  OutDataTypeStr=uint16
  Extract Bits : simulink/Logic and Bit Operations/Extract Bits  bitsToExtract=Range of bits  numBits=8  bitIdxRange=6  outScalingMode=Treat bit field as an integer
      settings: SourceProductName=Simulink
  Out1 : Outport
  wires:
  Data Type Conversion7/1 -> Out1/1
  In1/1 -> Extract Bits/1
  Extract Bits/1 -> Data Type Conversion7/1

== system DFADAS2_SenFus_v1_201204RC_training_210115/Signal Input (Input)/Signal Input (10ms) (Input10)/VehInfo/Vehicle Movement Signal Receive and Processing (VehMovRx)/VehSpd CAN Frame PreProcess (VehSpdCANFrmPPrcs)/CAN Diagnosis (CANDia)/CheckSum Diagnosis (ChkSumDia)/Bit Check(BChk)/Bit Operating (BOp)/ChksumPre3 ==
  In1 : Inport
  Data Type Conversion8 : DataTypeConversion  OutDataTypeStr=uint16
  Extract Bits1 : simulink/Logic and Bit Operations/Extract Bits  bitsToExtract=Range of bits  numBits=8  bitIdxRange=5  outScalingMode=Treat bit field as an integer
      settings: SourceProductName=Simulink
  Out1 : Outport
  wires:
  Data Type Conversion8/1 -> Out1/1
  In1/1 -> Extract Bits1/1
  Extract Bits1/1 -> Data Type Conversion8/1

== system DFADAS2_SenFus_v1_201204RC_training_210115/Signal Input (Input)/Signal Input (10ms) (Input10)/VehInfo/Vehicle Movement Signal Receive and Processing (VehMovRx)/VehSpd CAN Frame PreProcess (VehSpdCANFrmPPrcs)/CAN Diagnosis (CANDia)/CheckSum Diagnosis (ChkSumDia)/Bit Check(BChk)/Bit Operating (BOp)/ChksumPre4 ==
  In1 : Inport
  Data Type Conversion8 : DataTypeConversion  OutDataTypeStr=uint16
  Extract Bits1 : simulink/Logic and Bit Operations/Extract Bits  bitsToExtract=Range of bits  numBits=8  bitIdxRange=4  outScalingMode=Treat bit field as an integer
      settings: SourceProductName=Simulink
  Out1 : Outport
  wires:
  Extract Bits1/1 -> Data Type Conversion8/1
  In1/1 -> Extract Bits1/1
  Data Type Conversion8/1 -> Out1/1

== system DFADAS2_SenFus_v1_201204RC_training_210115/Signal Input (Input)/Signal Input (10ms) (Input10)/VehInfo/Vehicle Movement Signal Receive and Processing (VehMovRx)/VehSpd CAN Frame PreProcess (VehSpdCANFrmPPrcs)/CAN Diagnosis (CANDia)/CheckSum Diagnosis (ChkSumDia)/Bit Check(BChk)/Bit Operating (BOp)/ChksumPre5 ==
  In1 : Inport
  In2 : Inport  Port=2
  Add : Sum
  Data Type Conversion1 : DataTypeConversion  OutDataTypeStr=uint16
  Data Type Conversion4 : DataTypeConversion  OutDataTypeStr=uint16
  Shift Arithmetic2 : ArithShift  BitShiftNumber=-8
  Out1 : Outport
  wires:
  In1/1 -> Data Type Conversion4/1
  In2/1 -> Data Type Conversion1/1
  Shift Arithmetic2/1 -> Add/1
  Add/1 -> Out1/1
  Data Type Conversion4/1 -> Shift Arithmetic2/1
  Data Type Conversion1/1 -> Add/2

== system DFADAS2_SenFus_v1_201204RC_training_210115/Signal Input (Input)/Signal Input (10ms) (Input10)/VehInfo/Vehicle Movement Signal Receive and Processing (VehMovRx)/VehSpd CAN Frame PreProcess (VehSpdCANFrmPPrcs)/CAN Diagnosis (CANDia)/CheckSum Diagnosis (ChkSumDia)/Bit Check(BChk)/Bit Operating (BOp)/ChksumPre6 ==
  In1 : Inport
  In2 : Inport  Port=2
  Add : Sum
  Data Type Conversion1 : DataTypeConversion  OutDataTypeStr=uint16
  Data Type Conversion4 : DataTypeConversion  OutDataTypeStr=uint16
  Shift Arithmetic2 : ArithShift  BitShiftNumber=-8
  Out1 : Outport
  wires:
  Data Type Conversion1/1 -> Add/2
  Data Type Conversion4/1 -> Shift Arithmetic2/1
  Add/1 -> Out1/1
  Shift Arithmetic2/1 -> Add/1
  In2/1 -> Data Type Conversion1/1
  In1/1 -> Data Type Conversion4/1

== system DFADAS2_SenFus_v1_201204RC_training_210115/Signal Input (Input)/Signal Input (10ms) (Input10)/VehInfo/Vehicle Movement Signal Receive and Processing (VehMovRx)/VehSpd CAN Frame PreProcess (VehSpdCANFrmPPrcs)/CAN Diagnosis (CANDia)/CheckSum Diagnosis (ChkSumDia)/Bit Check(BChk)/Bit Operating (BOp)/ChksumPre7 ==
  In1 : Inport
  Data Type Conversion8 : DataTypeConversion  OutDataTypeStr=uint16
  Extract Bits1 : simulink/Logic and Bit Operations/Extract Bits  bitsToExtract=Range of bits  numBits=8  bitIdxRange=7  outScalingMode=Treat bit field as an integer
      settings: SourceProductName=Simulink
  Out1 : Outport
  wires:
  Data Type Conversion8/1 -> Out1/1
  In1/1 -> Extract Bits1/1
  Extract Bits1/1 -> Data Type Conversion8/1

== system DFADAS2_SenFus_v1_201204RC_training_210115/Signal Input (Input)/Signal Input (10ms) (Input10)/VehInfo/Vehicle Movement Signal Receive and Processing (VehMovRx)/Yaw State CAN Frame PreProcess (YawCANFrmPPrcs)/CAN Diagnosis (CANDia)/CheckSum Diagnosis (ChkSumDia)/Bit Check(BChk)/Bit Operating (BOp)/ChksumPre1 ==
  In1 : Inport
  Data Type Conversion7 : DataTypeConversion  OutDataTypeStr=uint16
  Out1 : Outport
  wires:
  In1/1 -> Data Type Conversion7/1
  Data Type Conversion7/1 -> Out1/1

== system DFADAS2_SenFus_v1_201204RC_training_210115/Signal Input (Input)/Signal Input (10ms) (Input10)/VehInfo/Vehicle Movement Signal Receive and Processing (VehMovRx)/Yaw State CAN Frame PreProcess (YawCANFrmPPrcs)/CAN Diagnosis (CANDia)/CheckSum Diagnosis (ChkSumDia)/Bit Check(BChk)/Bit Operating (BOp)/ChksumPre2 ==
  In1 : Inport
  Data Type Conversion7 : DataTypeConversion  OutDataTypeStr=uint16
  Extract Bits : simulink/Logic and Bit Operations/Extract Bits  bitsToExtract=Range of bits  numBits=8  bitIdxRange=6  outScalingMode=Treat bit field as an integer
      settings: SourceProductName=Simulink
  Out1 : Outport
  wires:
  Data Type Conversion7/1 -> Out1/1
  In1/1 -> Extract Bits/1
  Extract Bits/1 -> Data Type Conversion7/1

== system DFADAS2_SenFus_v1_201204RC_training_210115/Signal Input (Input)/Signal Input (10ms) (Input10)/VehInfo/Vehicle Movement Signal Receive and Processing (VehMovRx)/Yaw State CAN Frame PreProcess (YawCANFrmPPrcs)/CAN Diagnosis (CANDia)/CheckSum Diagnosis (ChkSumDia)/Bit Check(BChk)/Bit Operating (BOp)/ChksumPre3 ==
  In1 : Inport
  Data Type Conversion8 : DataTypeConversion  OutDataTypeStr=uint16
  Extract Bits1 : simulink/Logic and Bit Operations/Extract Bits  bitsToExtract=Range of bits  numBits=8  bitIdxRange=5  outScalingMode=Treat bit field as an integer
      settings: SourceProductName=Simulink
  Out1 : Outport
  wires:
  Data Type Conversion8/1 -> Out1/1
  In1/1 -> Extract Bits1/1
  Extract Bits1/1 -> Data Type Conversion8/1

== system DFADAS2_SenFus_v1_201204RC_training_210115/Signal Input (Input)/Signal Input (10ms) (Input10)/VehInfo/Vehicle Movement Signal Receive and Processing (VehMovRx)/Yaw State CAN Frame PreProcess (YawCANFrmPPrcs)/CAN Diagnosis (CANDia)/CheckSum Diagnosis (ChkSumDia)/Bit Check(BChk)/Bit Operating (BOp)/ChksumPre4 ==
  In1 : Inport
  Data Type Conversion8 : DataTypeConversion  OutDataTypeStr=uint16
  Extract Bits1 : simulink/Logic and Bit Operations/Extract Bits  bitsToExtract=Range of bits  numBits=8  bitIdxRange=4  outScalingMode=Treat bit field as an integer
      settings: SourceProductName=Simulink
  Out1 : Outport
  wires:
  Extract Bits1/1 -> Data Type Conversion8/1
  In1/1 -> Extract Bits1/1
  Data Type Conversion8/1 -> Out1/1

== system DFADAS2_SenFus_v1_201204RC_training_210115/Signal Input (Input)/Signal Input (10ms) (Input10)/VehInfo/Vehicle Movement Signal Receive and Processing (VehMovRx)/Yaw State CAN Frame PreProcess (YawCANFrmPPrcs)/CAN Diagnosis (CANDia)/CheckSum Diagnosis (ChkSumDia)/Bit Check(BChk)/Bit Operating (BOp)/ChksumPre5 ==
  In1 : Inport
  In2 : Inport  Port=2
  Add : Sum
  Data Type Conversion1 : DataTypeConversion  OutDataTypeStr=uint16
  Data Type Conversion4 : DataTypeConversion  OutDataTypeStr=uint16
  Shift Arithmetic2 : ArithShift  BitShiftNumber=-8
  Out1 : Outport
  wires:
  In1/1 -> Data Type Conversion4/1
  In2/1 -> Data Type Conversion1/1
  Shift Arithmetic2/1 -> Add/1
  Add/1 -> Out1/1
  Data Type Conversion4/1 -> Shift Arithmetic2/1
  Data Type Conversion1/1 -> Add/2

== system DFADAS2_SenFus_v1_201204RC_training_210115/Signal Input (Input)/Signal Input (10ms) (Input10)/VehInfo/Vehicle Movement Signal Receive and Processing (VehMovRx)/Yaw State CAN Frame PreProcess (YawCANFrmPPrcs)/CAN Diagnosis (CANDia)/CheckSum Diagnosis (ChkSumDia)/Bit Check(BChk)/Bit Operating (BOp)/ChksumPre6 ==
  In1 : Inport
  In2 : Inport  Port=2
  Add : Sum
  Data Type Conversion1 : DataTypeConversion  OutDataTypeStr=uint16
  Data Type Conversion4 : DataTypeConversion  OutDataTypeStr=uint16
  Shift Arithmetic2 : ArithShift  BitShiftNumber=-8
  Out1 : Outport
  wires:
  Data Type Conversion1/1 -> Add/2
  Data Type Conversion4/1 -> Shift Arithmetic2/1
  Add/1 -> Out1/1
  Shift Arithmetic2/1 -> Add/1
  In2/1 -> Data Type Conversion1/1
  In1/1 -> Data Type Conversion4/1

== system DFADAS2_SenFus_v1_201204RC_training_210115/Signal Input (Input)/Signal Input (10ms) (Input10)/VehInfo/Vehicle Movement Signal Receive and Processing (VehMovRx)/Yaw State CAN Frame PreProcess (YawCANFrmPPrcs)/CAN Diagnosis (CANDia)/CheckSum Diagnosis (ChkSumDia)/Bit Check(BChk)/Bit Operating (BOp)/ChksumPre7 ==
  In1 : Inport
  Data Type Conversion8 : DataTypeConversion  OutDataTypeStr=uint16
  Extract Bits1 : simulink/Logic and Bit Operations/Extract Bits  bitsToExtract=Range of bits  numBits=8  bitIdxRange=7  outScalingMode=Treat bit field as an integer
      settings: SourceProductName=Simulink
  Out1 : Outport
  wires:
  Data Type Conversion8/1 -> Out1/1
  In1/1 -> Extract Bits1/1
  Extract Bits1/1 -> Data Type Conversion8/1

== system DFADAS2_SenFus_v1_201204RC_training_210115/Signal Input (Input)/Signal Input (50ms) (Input50)/Cmr/CmrInfo/L0 Information (L0Info) /CAN Diagnosis (CANDia)1/CheckSum Diagnosis (ChkSumDia)/Bit Check(BChk)/Bit Operating (BOp)/ChksumPre1 ==
  In1 : Inport
  Data Type Conversion7 : DataTypeConversion  OutDataTypeStr=uint16
  Out1 : Outport
  wires:
  In1/1 -> Data Type Conversion7/1
  Data Type Conversion7/1 -> Out1/1

== system DFADAS2_SenFus_v1_201204RC_training_210115/Signal Input (Input)/Signal Input (50ms) (Input50)/Cmr/CmrInfo/L0 Information (L0Info) /CAN Diagnosis (CANDia)1/CheckSum Diagnosis (ChkSumDia)/Bit Check(BChk)/Bit Operating (BOp)/ChksumPre2 ==
  In1 : Inport
  Data Type Conversion7 : DataTypeConversion  OutDataTypeStr=uint16
  Extract Bits : simulink/Logic and Bit Operations/Extract Bits  bitsToExtract=Range of bits  numBits=8  bitIdxRange=6  outScalingMode=Treat bit field as an integer
      settings: SourceProductName=Simulink
  Out1 : Outport
  wires:
  Data Type Conversion7/1 -> Out1/1
  In1/1 -> Extract Bits/1
  Extract Bits/1 -> Data Type Conversion7/1

== system DFADAS2_SenFus_v1_201204RC_training_210115/Signal Input (Input)/Signal Input (50ms) (Input50)/Cmr/CmrInfo/L0 Information (L0Info) /CAN Diagnosis (CANDia)1/CheckSum Diagnosis (ChkSumDia)/Bit Check(BChk)/Bit Operating (BOp)/ChksumPre3 ==
  In1 : Inport
  Data Type Conversion8 : DataTypeConversion  OutDataTypeStr=uint16
  Extract Bits1 : simulink/Logic and Bit Operations/Extract Bits  bitsToExtract=Range of bits  numBits=8  bitIdxRange=5  outScalingMode=Treat bit field as an integer
      settings: SourceProductName=Simulink
  Out1 : Outport
  wires:
  Data Type Conversion8/1 -> Out1/1
  In1/1 -> Extract Bits1/1
  Extract Bits1/1 -> Data Type Conversion8/1

== system DFADAS2_SenFus_v1_201204RC_training_210115/Signal Input (Input)/Signal Input (50ms) (Input50)/Cmr/CmrInfo/L0 Information (L0Info) /CAN Diagnosis (CANDia)1/CheckSum Diagnosis (ChkSumDia)/Bit Check(BChk)/Bit Operating (BOp)/ChksumPre4 ==
  In1 : Inport
  Data Type Conversion8 : DataTypeConversion  OutDataTypeStr=uint16
  Extract Bits1 : simulink/Logic and Bit Operations/Extract Bits  bitsToExtract=Range of bits  numBits=8  bitIdxRange=4  outScalingMode=Treat bit field as an integer
      settings: SourceProductName=Simulink
  Out1 : Outport
  wires:
  Extract Bits1/1 -> Data Type Conversion8/1
  In1/1 -> Extract Bits1/1
  Data Type Conversion8/1 -> Out1/1

== system DFADAS2_SenFus_v1_201204RC_training_210115/Signal Input (Input)/Signal Input (50ms) (Input50)/Cmr/CmrInfo/L0 Information (L0Info) /CAN Diagnosis (CANDia)1/CheckSum Diagnosis (ChkSumDia)/Bit Check(BChk)/Bit Operating (BOp)/ChksumPre5 ==
  In1 : Inport
  In2 : Inport  Port=2
  Add : Sum
  Data Type Conversion1 : DataTypeConversion  OutDataTypeStr=uint16
  Data Type Conversion4 : DataTypeConversion  OutDataTypeStr=uint16
  Shift Arithmetic2 : ArithShift  BitShiftNumber=-8
  Out1 : Outport
  wires:
  In1/1 -> Data Type Conversion4/1
  In2/1 -> Data Type Conversion1/1
  Shift Arithmetic2/1 -> Add/1
  Add/1 -> Out1/1
  Data Type Conversion4/1 -> Shift Arithmetic2/1
  Data Type Conversion1/1 -> Add/2

== system DFADAS2_SenFus_v1_201204RC_training_210115/Signal Input (Input)/Signal Input (50ms) (Input50)/Cmr/CmrInfo/L0 Information (L0Info) /CAN Diagnosis (CANDia)1/CheckSum Diagnosis (ChkSumDia)/Bit Check(BChk)/Bit Operating (BOp)/ChksumPre6 ==
  In1 : Inport
  In2 : Inport  Port=2
  Add : Sum
  Data Type Conversion1 : DataTypeConversion  OutDataTypeStr=uint16
  Data Type Conversion4 : DataTypeConversion  OutDataTypeStr=uint16
  Shift Arithmetic2 : ArithShift  BitShiftNumber=-8
  Out1 : Outport
  wires:
  Data Type Conversion1/1 -> Add/2
  Data Type Conversion4/1 -> Shift Arithmetic2/1
  Add/1 -> Out1/1
  Shift Arithmetic2/1 -> Add/1
  In2/1 -> Data Type Conversion1/1
  In1/1 -> Data Type Conversion4/1

== system DFADAS2_SenFus_v1_201204RC_training_210115/Signal Input (Input)/Signal Input (50ms) (Input50)/Cmr/CmrInfo/L0 Information (L0Info) /CAN Diagnosis (CANDia)1/CheckSum Diagnosis (ChkSumDia)/Bit Check(BChk)/Bit Operating (BOp)/ChksumPre7 ==
  In1 : Inport
  Data Type Conversion8 : DataTypeConversion  OutDataTypeStr=uint16
  Extract Bits1 : simulink/Logic and Bit Operations/Extract Bits  bitsToExtract=Range of bits  numBits=8  bitIdxRange=7  outScalingMode=Treat bit field as an integer
      settings: SourceProductName=Simulink
  Out1 : Outport
  wires:
  Data Type Conversion8/1 -> Out1/1
  In1/1 -> Extract Bits1/1
  Extract Bits1/1 -> Data Type Conversion8/1

== system DFADAS2_SenFus_v1_201204RC_training_210115/Signal Input (Input)/Signal Input (50ms) (Input50)/Cmr/CmrInfo/L1 Information (L1Info)/CAN Diagnosis (CANDia)/CheckSum Diagnosis (ChkSumDia)/Bit Check(BChk)/Bit Operating (BOp)/ChksumPre1 ==
  In1 : Inport
  Data Type Conversion7 : DataTypeConversion  OutDataTypeStr=uint16
  Out1 : Outport
  wires:
  In1/1 -> Data Type Conversion7/1
  Data Type Conversion7/1 -> Out1/1

== system DFADAS2_SenFus_v1_201204RC_training_210115/Signal Input (Input)/Signal Input (50ms) (Input50)/Cmr/CmrInfo/L1 Information (L1Info)/CAN Diagnosis (CANDia)/CheckSum Diagnosis (ChkSumDia)/Bit Check(BChk)/Bit Operating (BOp)/ChksumPre2 ==
  In1 : Inport
  Data Type Conversion7 : DataTypeConversion  OutDataTypeStr=uint16
  Extract Bits : simulink/Logic and Bit Operations/Extract Bits  bitsToExtract=Range of bits  numBits=8  bitIdxRange=6  outScalingMode=Treat bit field as an integer
      settings: SourceProductName=Simulink
  Out1 : Outport
  wires:
  Data Type Conversion7/1 -> Out1/1
  In1/1 -> Extract Bits/1
  Extract Bits/1 -> Data Type Conversion7/1

== system DFADAS2_SenFus_v1_201204RC_training_210115/Signal Input (Input)/Signal Input (50ms) (Input50)/Cmr/CmrInfo/L1 Information (L1Info)/CAN Diagnosis (CANDia)/CheckSum Diagnosis (ChkSumDia)/Bit Check(BChk)/Bit Operating (BOp)/ChksumPre3 ==
  In1 : Inport
  Data Type Conversion8 : DataTypeConversion  OutDataTypeStr=uint16
  Extract Bits1 : simulink/Logic and Bit Operations/Extract Bits  bitsToExtract=Range of bits  numBits=8  bitIdxRange=5  outScalingMode=Treat bit field as an integer
      settings: SourceProductName=Simulink
  Out1 : Outport
  wires:
  Data Type Conversion8/1 -> Out1/1
  In1/1 -> Extract Bits1/1
  Extract Bits1/1 -> Data Type Conversion8/1
